simulink model "Bebop_sim_joystick_freeflight"  (R2018a)
settings: Solver=VariableStepAuto  StartTime=0.0  StopTime=30  RelTol=1e-3
libraries: vrlib x1
settings Model: EnablePacing=on  Creator=derek  LastModifiedBy=vinni

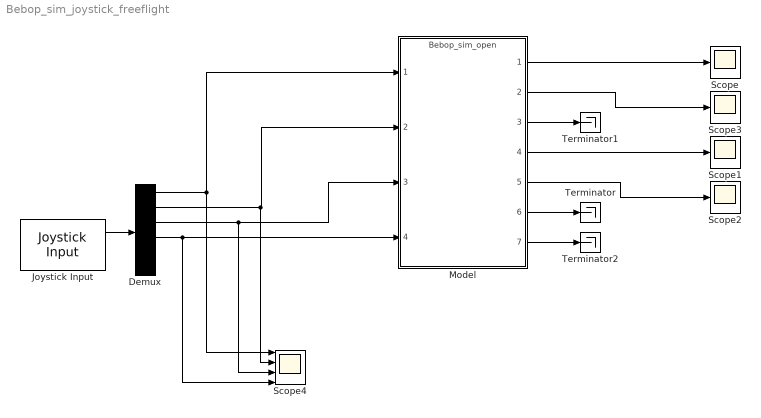
== system Bebop_sim_joystick_freeflight ==
  Demux : Demux  Outputs=6
  Joystick Input : vrlib/Joystick Input  joyid=1  adjustports=on  forcefeed=off
      settings: SourceProductBaseCode=VR
  Model : ModelReference  ModelNameDialog=Bebop_sim_open.slx  SimulationMode=Normal  ModelReferenceVersion=1.13
  Scope{,1..3} (4 alike) : Scope
  Scope4 : Scope  NumInputPorts=4
  Terminator : Terminator
  Terminator1 : Terminator
  Terminator2 : Terminator
  wires:
  Demux/1 -> Model/1, Scope4/1
  Demux/2 -> Model/2, Scope4/2
  Demux/3 -> Model/3, Scope4/3
  Model/1 -> Scope/1
  Model/4 -> Scope1/1
  Model/5 -> Scope2/1
  Model/2 -> Scope3/1
  Model/7 -> Terminator2/1
  Model/6 -> Terminator/1
  Model/3 -> Terminator1/1
  Demux/4 -> Model/4, Scope4/4
  Joystick Input/1 -> Demux/1
